simulink model "q3a3576b"  (Simulink 7.7)
settings: Solver=ode45  StartTime=0.0  StopTime=10.0  RelTol=1e-3
libraries: simulink x1
settings Model: Creator=Owner  LastModifiedBy=Owner

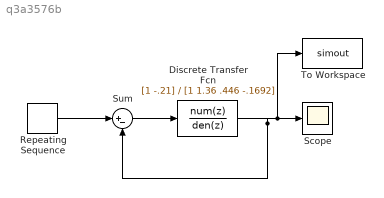
== system q3a3576b ==
  Discrete Transfer Fcn : DiscreteTransferFcn  Numerator=[1 -.21]  Denominator=[1 1.36 .446 -.1692]
  Repeating Sequence : simulink/Sources/Repeating Sequence  SystemSampleTime=-1  rep_seq_t=[0:.002:.1]  rep_seq_y=[.21.^[1:1:51]]
  Scope : Scope
  Sum : Sum  Inputs=|+-
  To Workspace : ToWorkspace  VariableName=simout  SampleTime=-1  SaveFormat=Structure
  wires:
  Repeating Sequence/1 -> Sum/1
  Sum/1 -> Discrete Transfer Fcn/1
  Discrete Transfer Fcn/1 -> Sum/2, Scope/1, To Workspace/1
